simulink model "ADC_personal"  (R2024a)
settings: Solver=FixedStepAuto  StartTime=0.0  StopTime=600e-06  FixedStep=1/250e6  RelTol=1e-3
PreLoadFcn:
  | jitter = 145e-15;
  | nonlingain = 0.17;
StopFcn:
  | dy = out.yout - mean(out.yout);
  | rmsjitter = std(dy);
  | histogram(dy,50);
  | title(['\bfjitter didtribution: RMS jitter = ',num2str(rmsjitter),'s']);
  | xlabel('Time (s) -->');
  | ylabel('Occurances (count) -->');
libraries: dspfdesign x2
settings Model: Creator=GILBERT KELECHI  LastModifiedBy=GILBERT KELECHI
settings DataIOCC: LimitDataPoints=on  MaxDataPoints=200000  SaveFormat=Array
settings DebuggingCC: SingleTaskRateTransMsg=error
settings HardwareCC: ProdBitPerPointer=32  ProdBitPerSizeT=32  ProdBitPerPtrDiffT=32  ProdLargestAtomicFloat=None  ProdWordSize=32  ProdHWDeviceType=Altera->SoC (ARM Cortex A)  TargetBitPerPointer=64  TargetBitPerSizeT=64  TargetBitPerPtrDiffT=64  TargetLongLongMode=on  TargetIntDivRoundTo=Zero  TargetEndianess=LittleEndian  TargetWordSize=64  TargetHWDeviceType=Custom Processor->MATLAB Host Computer  ProdEqTarget=off
settings RTWCC: GenCodeOnly=on

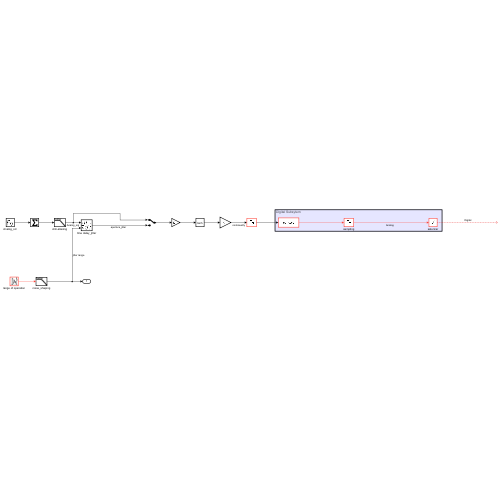
[thumbnail: Simulink's stored preview of the top-level diagram]
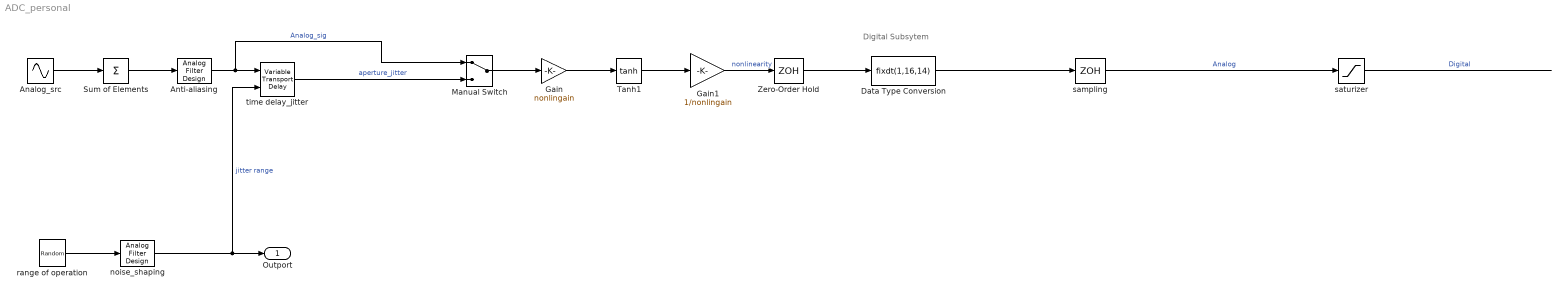
== system ADC_personal ==
  note: Digital Subsytem
  Analog_src : Sin  Amplitude=0.5  Frequency=2*pi*20e6  SampleTime=0
  Anti-aliasing : dspfdesign/Analog Filter Design  method=Butterworth  filttype=Lowpass  N=8  Wlo=2*pi*125e6  Whi=80  Rp=2  Rs=40
  Data Type Conversion : DataTypeConversion  OutDataTypeStr=fixdt(1,16,14)  SaturateOnIntegerOverflow=off  RndMeth=Floor
  Gain : Gain  Gain=nonlingain
  Gain1 : Gain  Gain=1/nonlingain
  Manual Switch : ManualSwitch
  Sum of Elements : Sum  Inputs=+
  Tanh1 : Trigonometry  Operator=tanh
  Zero-Order Hold : ZeroOrderHold  SampleTime=1/250e6
  noise_shaping : dspfdesign/Analog Filter Design  method=Butterworth  filttype=Lowpass  N=3  Wlo=2*pi*20e6  Whi=80  Rp=2  Rs=40
  range of operation : UniformRandomNumber  Minimum=0  Maximum=10.36*sqrt(12)*jitter  Seed=1234  SampleTime=0
  sampling : ZeroOrderHold  SampleTime=1/250e6
  saturizer : Saturate
  time delay_jitter : VariableTransportDelay  MaximumDelay=10e-12  ZeroDelay=on  TransDelayFeedthrough=on
  Outport : Outport
  wires:
  Analog_src/1 -> Sum of Elements/1
  range of operation/1 -> noise_shaping/1
  noise_shaping/1 -> Outport/1, time delay_jitter/2  "jitter range"
  time delay_jitter/1 -> Manual Switch/2  "aperture_jitter"
  Sum of Elements/1 -> Anti-aliasing/1
  Anti-aliasing/1 -> Manual Switch/1, time delay_jitter/1  "Analog_sig"
  Gain/1 -> Tanh1/1
  Tanh1/1 -> Gain1/1
  Manual Switch/1 -> Gain/1
  Gain1/1 -> Zero-Order Hold/1  "nonlinearity"
  saturizer/1 -> ?  "Digital"
  Zero-Order Hold/1 -> Data Type Conversion/1
  Data Type Conversion/1 -> sampling/1
  sampling/1 -> saturizer/1  "Analog"
